simulink model "voltameter_Arduino"  (R2023b)
settings: Solver=FixedStepDiscrete  StartTime=0.0  StopTime=inf  FixedStep=0.01  RelTol=1e-3
libraries: arduinolib x1
settings Model: ExtModeTrigDuration=2  Creator=OS 10  LastModifiedBy=OS 10
settings OptimizationCC: DefaultParameterBehavior=Inlined  GainParamInheritBuiltInType=on  UseSpecifiedMinMax=on  InlineInvariantSignals=on  EnhancedBackFolding=on  BooleansAsBitfields=on  PassReuseOutputArgsAs=Individual arguments  StateBitsets=on  DataBitsets=on  ZeroExternalMemoryAtStartup=off  ZeroInternalMemoryAtStartup=off  MaxStackSize=64  OptimizeBlockOrder=speed  DifferentSizesBufferReuse=on  EfficientTunableParamExpr=on
settings DebuggingCC: ParameterTunabilityLossMsg=error
settings HardwareCC: ProdBitPerInt=16  ProdBitPerPointer=16  ProdBitPerSizeT=16  ProdBitPerPtrDiffT=16  ProdLargestAtomicFloat=None  ProdWordSize=8  ProdHWDeviceType=Atmel->AVR
settings SFSimCC: MATLABDynamicMemAlloc=off
settings RTWCC: Description=Embedded Coder  SystemTargetFile=ert.tlc  HardwareBoard=Arduino Uno  TemplateMakefile=ert_default_tmf  Toolchain=Arduino AVR  BuildConfiguration=Faster Runs
settings CodeAppCC: ForceParamTrailComments=on  IgnoreCustomStorageClasses=off  OperatorAnnotations=on  SimulinkDataObjDesc=on  SFDataObjDesc=on  InsertBlockDesc=on
settings ERTTargetCC: CombineSignalStateStructs=on  SuppressErrorStatus=on  SupportContinuousTime=on  SupportVariableSizeSignals=on  ExtModeTransport=3  ExtModeStaticAlloc=on  ExtModeAutomaticAllocSize=off  ExtModeStaticAllocSize=250  ExtModeMexFile=ext_xcp  ExtModeIntrfLevel=Level2 - Open

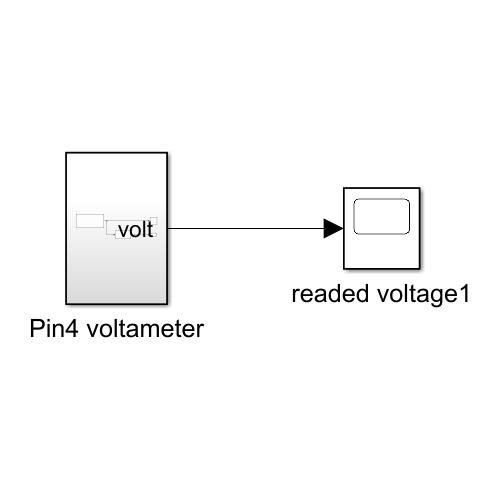
[thumbnail: Simulink's stored preview of the top-level diagram]
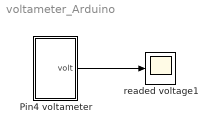
== system voltameter_Arduino ==
  Pin4 voltameter : Subsystem
  readed voltage1 : Scope
  wires:
  Pin4 voltameter/1("volt ") -> readed voltage1/1

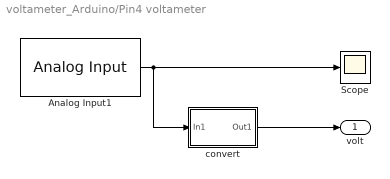
== system voltameter_Arduino/Pin4 voltameter ==
  Analog Input1 : arduinolib/Analog Input  pinNumber=4  ReadResultsOnly=off  ConversionTriggerSource=Software  ExternalTriggerType=uint32( 0 )  OutputDataType=uint16  EnableConversionCompleteNotify=off  EnableOuputStatus=off  SampleTime=0.01  blockPlatform=arduino
  Scope : Scope
  convert : Subsystem
  "volt " : Outport
  wires:
  Analog Input1/1 -> convert/1(In1), Scope/1
  convert/1(Out1) -> "volt "/1

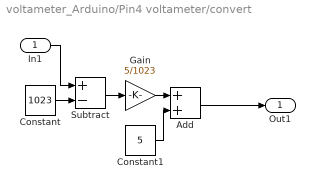
== system voltameter_Arduino/Pin4 voltameter/convert ==
  In1 : Inport
  Add : Sum
  Constant : Constant  Value=1023
  Constant1 : Constant  Value=5
  Gain : Gain  Gain=5/1023
  Subtract : Sum  Inputs=+-
  Out1 : Outport
  wires:
  Gain/1 -> Add/1
  Subtract/1 -> Gain/1
  Constant/1 -> Subtract/2
  Constant1/1 -> Add/2
  Add/1 -> Out1/1
  In1/1 -> Subtract/1
